simulink model "FIR_filter_model"  (R2020b)
settings: Solver=FixedStepAuto  StartTime=0.0  StopTime=30  FixedStep=0.6  RelTol=1e-3
settings Model: Creator=153  LastModifiedBy=153
settings DataIOCC: SaveOutput=off  SaveTime=off

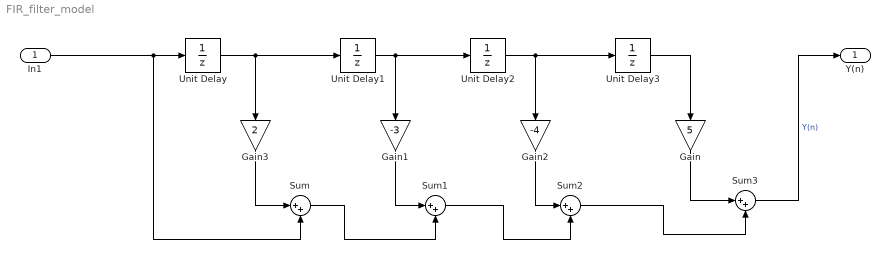
== system FIR_filter_model ==
  In1 : Inport  OutDataTypeStr=double  PortDimensions=1  SampleTime=[0.59999999999999998,0]
  Gain : Gain  Gain=5
  Gain1 : Gain  Gain=-3
  Gain2 : Gain  Gain=-4
  Gain3 : Gain  Gain=2
  Sum{,1..3} (4 alike) : Sum  Inputs=|++
  Unit Delay{,1..3} (4 alike) : UnitDelay  SampleTime=-1  HasFrameUpgradeWarning=on
  Y(n) : Outport  OutDataTypeStr=double  PortDimensions=1  SampleTime=[0.59999999999999998,0]
  wires:
  Gain3/1 -> Sum/1
  Sum1/1 -> Sum2/2
  Unit Delay2/1 -> Gain2/1, Unit Delay3/1
  Sum/1 -> Sum1/2
  Gain1/1 -> Sum1/1
  Unit Delay/1 -> Unit Delay1/1, Gain3/1
  Gain2/1 -> Sum2/1
  In1/1 -> Unit Delay/1, Sum/2
  Unit Delay1/1 -> Gain1/1, Unit Delay2/1
  Gain/1 -> Sum3/1
  Sum2/1 -> Sum3/2
  Unit Delay3/1 -> Gain/1
  Sum3/1 -> Y(n)/1  "Y(n)"
